simulink model "FMUEngine"  (R2026b)
settings: Solver=VariableStepAuto
undefined symbols (not defined in the file): Afr, BSFC, CrkAng, EngSpdOut, EngTrq, ExhManGasTemp, FuelFlw, FuelVolFlw, IntkPortFlw, NormAirChrg, PlntEngFuelSg
libraries: autolibsharedcommon x1, simulink_extras x1, autolibpowerinfoutils x1, autolibutils x1
settings Model: ModifiedByFormat=The MathWorks, Inc.  Creator=The MathWorks, Inc.  LastModifiedBy=The MathWorks, Inc.
settings OptimizationCC: ReuseModelBlockBuffer=off
settings DebuggingCC: SubsystemReferenceDiagnosticForUnitTest=warning

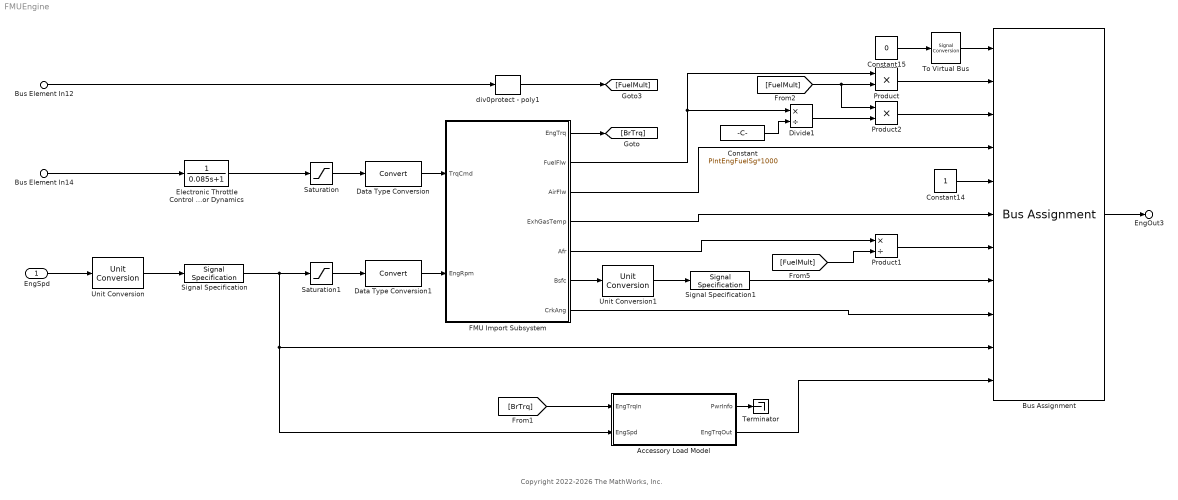
== system FMUEngine ==
  note: Copyright 2022-2026 The MathWorks, Inc.
  EngSpd : Inport  Unit=rad/sec
  Bus Element In12 : Inport  Port=2  PortName=Cntrl  Element=Engine.ClsdLpFuelMult
  Bus Element In14 : Inport  Port=2  PortName=Cntrl  Element=Engine.TrqCmd
  Accessory Load Model : Subsystem
  Bus Assignment : BusAssignment  AssignedSignals=FuelFlw,FuelVolFlw,IntkPortFlw,NormAirChrg,ExhManGasTemp,Afr,BSFC,CrkAng,EngSpdOut,EngTrq
  Constant : Constant  Value=PlntEngFuelSg*1000  SampleTime=-1
  Constant14 : Constant  SampleTime=-1
  Constant15 : Constant  Value=0  OutDataTypeStr=Bus: EngineBUS  SampleTime=Inf
  Data Type Conversion : DataTypeConversion  SaturateOnIntegerOverflow=off  RndMeth=Floor
  Data Type Conversion1 : DataTypeConversion  SaturateOnIntegerOverflow=off  RndMeth=Floor
  Divide1 : Product  Inputs=*/
  Electronic Throttle Control Actuator Dynamics : TransferFcn  Denominator=[0.085 1]
  FMU Import Subsystem : Subsystem
  Product : Product
  Product1 : Product  Inputs=*/
  Product2 : Product
  Saturation : Saturate  UpperLimit=inf  LowerLimit=0  ZeroCross=off
  Saturation1 : Saturate  UpperLimit=inf  LowerLimit=0  ZeroCross=off
  Signal Specification : SignalSpecification  Unit=rpm
  Signal Specification1 : SignalSpecification  Unit=g/kW/hr
  Terminator : Terminator
  To Virtual Bus : SignalConversion  ConversionOutput=Virtual bus  OverrideOpt=off
  Unit Conversion : UnitConversion
  Unit Conversion1 : UnitConversion
  div0protect - poly1 : autolibutils/div0protect - poly  thresh=0.01  ZeroCross1=off  aMode=aMode
  EngOut3 : Outport  PortName=EngFdbk
  wires:
  Signal Specification/1 -> Saturation1/1, Accessory Load Model/2(EngSpd), Bus Assignment/10
  FMU Import Subsystem/5(Afr) -> Product1/1
  Constant14/1 -> Bus Assignment/5
  FMU Import Subsystem/2(FuelFlw) -> Product/1, Divide1/1
  Constant/1 -> Divide1/2
  [BrTrq] -> Accessory Load Model/1(EngTrqIn)
  Product/1 -> Bus Assignment/2
  EngSpd/1 -> Unit Conversion/1
  Accessory Load Model/2(EngTrqOut) -> Bus Assignment/11
  Unit Conversion/1 -> Signal Specification/1
  Bus Element In12/1 -> div0protect - poly1/1
  Product2/1 -> Bus Assignment/3
  Product1/1 -> Bus Assignment/7
  Accessory Load Model/1(PwrInfo) -> Terminator/1
  FMU Import Subsystem/1(EngTrq) -> [BrTrq]
  FMU Import Subsystem/3(AirFlw) -> Bus Assignment/4
  FMU Import Subsystem/4(ExhGasTemp) -> Bus Assignment/6
  FMU Import Subsystem/6(Bsfc) -> Unit Conversion1/1
  FMU Import Subsystem/7(CrkAng) -> Bus Assignment/9
  To Virtual Bus/1 -> Bus Assignment/1
  Constant15/1 -> To Virtual Bus/1
  Bus Assignment/1 -> EngOut3/1
  div0protect - poly1/1 -> [FuelMult]
  [FuelMult] -> Product1/2
  [FuelMult] -> Product2/1, Product/2
  Divide1/1 -> Product2/2
  Signal Specification1/1 -> Bus Assignment/8
  Unit Conversion1/1 -> Signal Specification1/1
  Saturation1/1 -> Data Type Conversion1/1
  Data Type Conversion1/1 -> FMU Import Subsystem/2(EngRpm)
  Saturation/1 -> Data Type Conversion/1
  Data Type Conversion/1 -> FMU Import Subsystem/1(TrqCmd)
  Bus Element In14/1 -> Electronic Throttle Control Actuator Dynamics/1
  Electronic Throttle Control Actuator Dynamics/1 -> Saturation/1

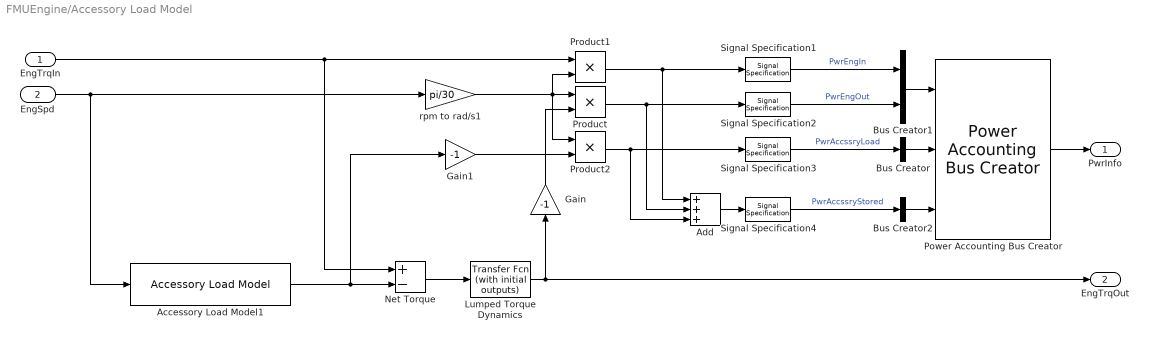
== system FMUEngine/Accessory Load Model ==
  EngTrqIn : Inport
  EngSpd : Inport  Port=2
  Accessory Load Model1 : autolibsharedcommon/Accessory Load Model  AccPwrTbl=PlntEngAccPwrTbl  AccSpdBpts=PlntEngAccSpdBpt  aMode=aMode
  Add : Sum  Inputs=+++
  Bus Creator : BusCreator  Inputs=1
  Bus Creator1 : BusCreator  Inputs=2
  Bus Creator2 : BusCreator  Inputs=1
  Gain : Gain  Gain=-1
  Gain1 : Gain  Gain=-1
  Lumped Torque Dynamics : simulink_extras/Additional Linear/Transfer Fcn (with initial outputs)  N=[1]  D=[0.2 1]  Y0=PlntEngInitTrq  U0=0
  Net Torque : Sum  Inputs=+-
  Power Accounting Bus Creator : autolibpowerinfoutils/Power Accounting Bus Creator  AssctBlkSelPopup=Parent  RefBlkName='libraryname/blkname'  PwrTrnsfrdCheckBox=on  PwrNotTrnsfrdCheckBox=on  PwrStoredCheckBox=on  aMode=1
      settings: LibrarySourceBlock=autolibpowerutils/Power Accounting Bus Creator
  Product : Product
  Product1 : Product
  Product2 : Product
  Signal Specification{1..4} (4 alike) : SignalSpecification  Unit=W
  rpm to rad/s1 : Gain  Gain=pi/30
  PwrInfo : Outport  VectorParamsAs1DForOutWhenUnconnected=off
  EngTrqOut : Outport  Port=2  Unit=N*m  VectorParamsAs1DForOutWhenUnconnected=off
  wires:
  Product1/1 -> Signal Specification1/1, Add/1
  Add/1 -> Signal Specification4/1
  Signal Specification3/1 -> Bus Creator/1  "PwrAccssryLoad"
  Signal Specification4/1 -> Bus Creator2/1  "PwrAccssryStored"
  Bus Creator2/1 -> Power Accounting Bus Creator/3
  Gain1/1 -> Product2/2
  Gain/1 -> Product/2
  Signal Specification2/1 -> Bus Creator1/2  "PwrEngOut"
  Signal Specification1/1 -> Bus Creator1/1  "PwrEngIn"
  rpm to rad/s1/1 -> Product/1, Product2/1, Product1/2
  Product/1 -> Signal Specification2/1, Add/2
  Power Accounting Bus Creator/1 -> PwrInfo/1
  Product2/1 -> Signal Specification3/1, Add/3
  EngTrqIn/1 -> Net Torque/1, Product1/1
  Bus Creator1/1 -> Power Accounting Bus Creator/1
  Bus Creator/1 -> Power Accounting Bus Creator/2
  Net Torque/1 -> Lumped Torque Dynamics/1
  Lumped Torque Dynamics/1 -> Gain/1, EngTrqOut/1
  EngSpd/1 -> Accessory Load Model1/1, rpm to rad/s1/1
  Accessory Load Model1/1 -> Net Torque/2, Gain1/1

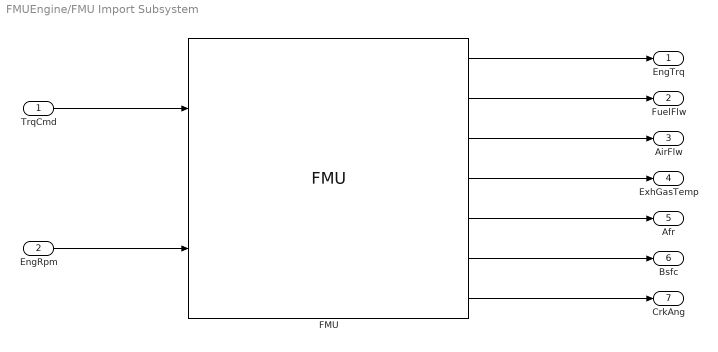
== system FMUEngine/FMU Import Subsystem ==
  TrqCmd : Inport  Description=Commanded brake torque  Unit=N*m
  EngRpm : Inport  Description=Engine speed in rpm  Port=2  Unit=rev/min
  FMU : FMU  FMUName=VvcFmuEngEx.fmu  FMUMode=CoSimulation  FMUSampleTime=0.03  FMUCreateBusObject=off  FMUInitializeEnumObject=off  PlntEngBsfcAvg=350  mask(VvcFmuEngEx [Co-Simulation, v2.0]){}
      mask Display:
      | disp('VvcFmuEngEx');
      | port_label('output',1,'EngTrq');
      | port_label('output',2,'FuelFlw');
      | port_label('output',3,'AirFlw');
      | port_label('output',4,'ExhGasTemp');
      | port_label('output',5,'Afr');
      | port_label('output',6,'Bsfc');
      | port_label('output',7,'CrkAng');
      | port_label('input',1,'TrqCmd');
      | port_label('input',2,'EngRpm');
  EngTrq : Outport  Description=Brake torque  Unit=N*m
  FuelFlw : Outport  Description=Fuel mass flow rate  Port=2  Unit=kg/s
  AirFlw : Outport  Description=Air mass flow rate  Port=3  Unit=kg/s
  ExhGasTemp : Outport  Description=Exhaust gas temperature  Port=4  Unit=K
  Afr : Outport  Description=Air fuel ratio  Port=5  Unit=1
  Bsfc : Outport  Description=Brake specific fuel consumption  Port=6
  CrkAng : Outport  Description=Crank angle  Port=7  Unit=deg
  wires:
  TrqCmd/1 -> FMU/1
  EngRpm/1 -> FMU/2
  FMU/1 -> EngTrq/1
  FMU/2 -> FuelFlw/1
  FMU/3 -> AirFlw/1
  FMU/4 -> ExhGasTemp/1
  FMU/5 -> Afr/1
  FMU/6 -> Bsfc/1
  FMU/7 -> CrkAng/1
